simulink model "Resistor_system"  (R2024b)
settings: Solver=VariableStepAuto  StartTime=0.0  StopTime=10.0  RelTol=1e-3
model workspace (MAT data in the model file):
  R = Simulink.Parameter
  R.Value = 1000000
  R.Complexity = 'real'
  R.Dimensions = [1 1]
  R.DataType = 'auto'
settings Model: Creator=omari  LastModifiedBy=omari

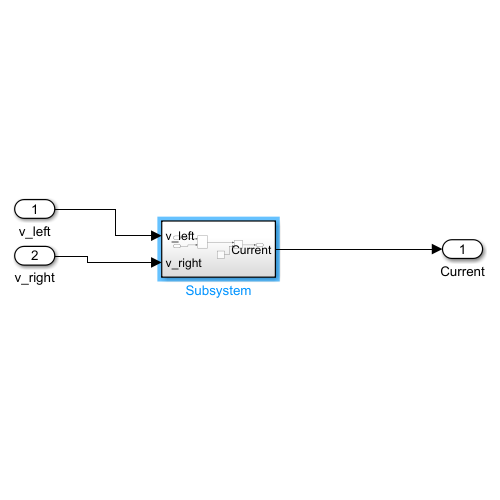
[thumbnail: Simulink's stored preview of the top-level diagram]
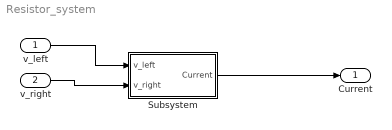
== system Resistor_system ==
  v_left : Inport
  v_right : Inport  Port=2
  Subsystem : Subsystem
  Current : Outport
  wires:
  v_left/1 -> Subsystem/1(v_left)
  v_right/1 -> Subsystem/2(v_right)
  Subsystem/1(Current) -> Current/1

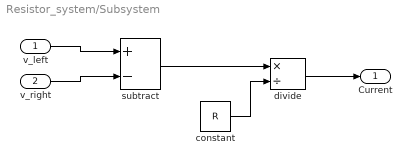
== system Resistor_system/Subsystem ==
  v_left : Inport
  v_right : Inport  Port=2
  constant : Constant  Value=R
  divide : Product  Inputs=*/
  subtract : Sum  Inputs=+-
  Current : Outport
  wires:
  divide/1 -> Current/1
  v_left/1 -> subtract/1
  constant/1 -> divide/2
  v_right/1 -> subtract/2
  subtract/1 -> divide/1
